simulink model "vehicle"  (R2024a)
settings: Solver=VariableStepAuto  StartTime=0.0  StopTime=10.0  RelTol=1e-3
values from neighbouring files (symbols this model uses):
  A = 2.2    [vehicle_params.m]
  Cd = 0.3    [vehicle_params.m]
  Cr = 0.015    [vehicle_params.m]
  efficiency = 0.88    [vehicle_params.m]
  g = 9.81    [vehicle_params.m]
  gear_ratio = 8    [vehicle_params.m]
  m = 1500    [vehicle_params.m]
  rho = 1.225    [vehicle_params.m]
  road_slope_deg = 0    [vehicle_params.m]
  rpm_breakpoints = [0 1000 2000 3000 4000 5000 6000 7000]    [vehicle_params.m]
  torque_data = [0  80   140  170  180  160  120  60]    [vehicle_params.m]
  wheel_radius = 0.3    [vehicle_params.m]
settings Model: Creator=khali  LastModifiedBy=khali

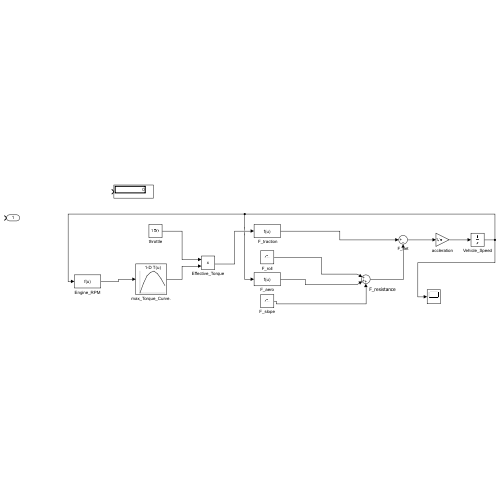
[thumbnail: Simulink's stored preview of the top-level diagram]
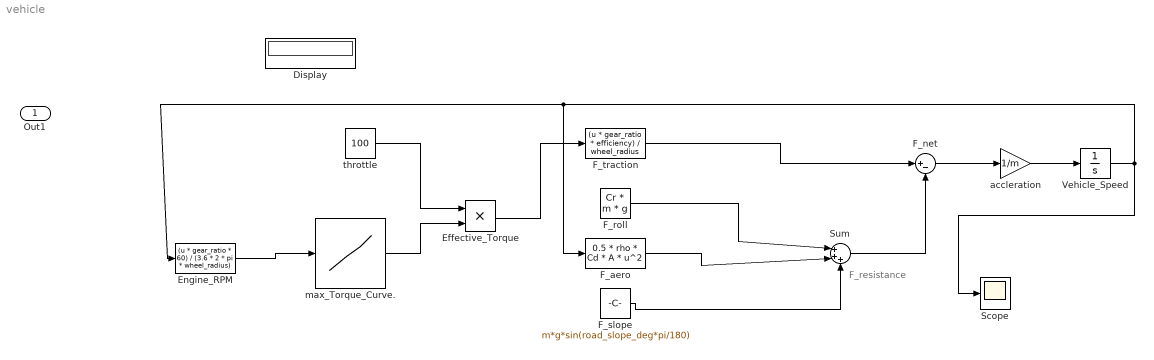
== system vehicle ==
  note: F_resistance
  " F_traction" : Fcn  Expr=(u * gear_ratio * efficiency) / wheel_radius
  Display : Display
  Effective_Torque : Product
  Engine_RPM : Fcn  Expr=(u * gear_ratio * 60) / (3.6 * 2 * pi * wheel_radius)
  F_aero : Fcn  Expr=0.5 * rho * Cd * A * u^2
  F_net : Sum  Inputs=|+-
  F_roll : Constant  Value=Cr * m * g
  F_slope : Constant  Value=m*g*sin(road_slope_deg*pi/180)
  Scope : Scope
  Sum : Sum  Inputs=|+++
  Vehicle_Speed : Integrator  InitialCondition=120
  accleration : Gain  Gain=1/m
  max_Torque_Curve. : Lookup_n-D  NumberOfTableDimensions=1  BreakpointsForDimension1=rpm_breakpoints  Table=torque_data  InternalRulePriority=Speed  RndMeth=Simplest
  throttle : Constant  Value=100
  Out1 : Outport
  wires:
  F_aero/1 -> Sum/2
  F_slope/1 -> Sum/3
  Sum/1 -> F_net/2
  F_net/1 -> accleration/1
  accleration/1 -> Vehicle_Speed/1
  Effective_Torque/1 -> " F_traction"/1
  throttle/1 -> Effective_Torque/1
  max_Torque_Curve./1 -> Effective_Torque/2
  Engine_RPM/1 -> max_Torque_Curve./1
  " F_traction"/1 -> F_net/1
  F_roll/1 -> Sum/1
  Vehicle_Speed/1 -> Engine_RPM/1, F_aero/1, Scope/1
